simulink model "T_model_2"  (Simulink 7.2)
settings: Solver=ode23t  StartTime=0.0  StopTime=0.1  RelTol=1e-6
libraries: powerlib x19, powerlib_extras x5, srolib x3
settings Model: Creator=user  LastModifiedBy=user

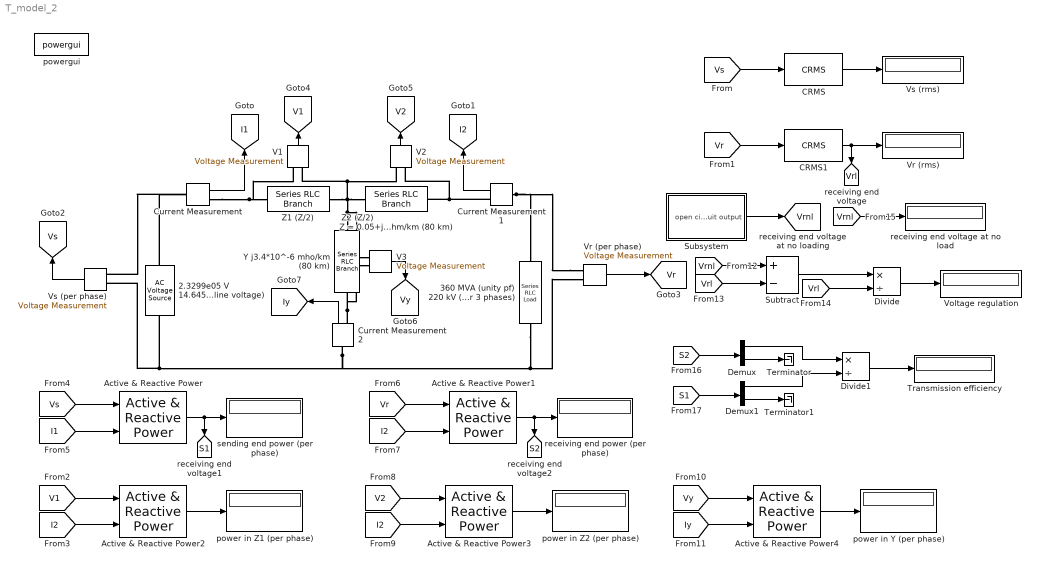
== system T_model_2 ==
  2.3299e05 V 14.64579 deg (line voltage) : powerlib/Electrical Sources/AC Voltage Source  Orientation=up  DialogController=POWERSYS.PowerSysDialog  SystemSampleTime=-1  Amplitude=(1.34526e5)*1.414  Phase=14.64579  Frequency=60  SampleTime=-1  Measurements=Voltage
  360 MVA (unity pf) 220 kV (rms) (for 3 phases) : powerlib/Elements/Series RLC Load  Orientation=down  DialogController=POWERSYS.PowerSysDialog  PhysicalDomain=powersysdomain  SubClassName=unknown  LeftPortType=p1  RightPortType=p1  LConnTagsString=a  RConnTagsString=__new0  NominalVoltage=220000/1.732  NominalFrequency=60  ActivePower=(360e6)/3  InductivePower=0  CapacitivePower=0  Setx0=off  InitialVoltage=0  SetiL0=off  InitialCurrent=0  Measurements=Branch voltage and current
  Active & Reactive Power{,1..4} (5 alike) : powerlib_extras/Measurements/Active & Reactive Power  DialogController=POWERSYS.PowerSysDialog  SystemSampleTime=-1  f1=60
  CRMS : srolib/RMS Blocks/CRMS  SystemSampleTime=-1
  CRMS1 : srolib/RMS Blocks/CRMS  SystemSampleTime=-1
  Current Measurement : powerlib/Measurements/Current Measurement  DialogController=POWERSYS.PowerSysDialog  SystemSampleTime=-1  PhasorSimulation=off  OutputType=Complex  PSBequivalent=0
  Current Measurement1 : powerlib/Measurements/Current Measurement  Orientation=left  DialogController=POWERSYS.PowerSysDialog  SystemSampleTime=-1  PhasorSimulation=off  OutputType=Complex  PSBequivalent=0
  Current Measurement2 : powerlib/Measurements/Current Measurement  Orientation=up  DialogController=POWERSYS.PowerSysDialog  SystemSampleTime=-1  PhasorSimulation=off  OutputType=Complex  PSBequivalent=0
  Demux : Demux  Outputs=2
  Demux1 : Demux  Outputs=2
  Divide : Product  Inputs=*/  OutDataType=sfix(16)  OutScaling=2^-10
  Divide1 : Product  Inputs=*/  OutDataType=sfix(16)  OutScaling=2^-10
  Subsystem : Subsystem
  Subtract : Sum  Inputs=+-  OutDataType=sfix(16)  OutScaling=2^-10
  Terminator : Terminator
  Terminator1 : Terminator
  Transmission efficiency : Display
  V1 : powerlib/Measurements/Voltage Measurement  Orientation=up  DialogController=POWERSYS.PowerSysDialog  SystemSampleTime=-1  PhasorSimulation=off  OutputType=Complex  PSBequivalent=0
  V2 : powerlib/Measurements/Voltage Measurement  Orientation=up  DialogController=POWERSYS.PowerSysDialog  SystemSampleTime=-1  PhasorSimulation=off  OutputType=Complex  PSBequivalent=0
  V3 : powerlib/Measurements/Voltage Measurement  DialogController=POWERSYS.PowerSysDialog  SystemSampleTime=-1  PhasorSimulation=off  OutputType=Complex  PSBequivalent=0
  Voltage regulation : Display
  Vr (per phase) : powerlib/Measurements/Voltage Measurement  DialogController=POWERSYS.PowerSysDialog  SystemSampleTime=-1  PhasorSimulation=off  OutputType=Complex  PSBequivalent=0
  Vr (rms) : Display
  Vs (per phase) : powerlib/Measurements/Voltage Measurement  Orientation=left  DialogController=POWERSYS.PowerSysDialog  SystemSampleTime=-1  PhasorSimulation=off  OutputType=Complex  PSBequivalent=0
  Vs (rms) : Display
  Y j3.4*10^-6 mho/km (80 km) : powerlib/Elements/Series RLC Branch  Orientation=down  DialogController=POWERSYS.PowerSysDialog  PhysicalDomain=powersysdomain  SubClassName=unknown  LeftPortType=p1  RightPortType=p1  LConnTagsString=__new0  RConnTagsString=__new0  BranchType=C  Resistance=1  Inductance=1e-3  SetiL0=off  InitialCurrent=0  Capacitance=80*(3.4e-6)/(120*3.14)  Setx0=off  InitialVoltage=0  Measurements=Branch voltage and current
  Z1 (Z/2) : powerlib/Elements/Series RLC Branch  DialogController=POWERSYS.PowerSysDialog  PhysicalDomain=powersysdomain  SubClassName=unknown  LeftPortType=p1  RightPortType=p1  LConnTagsString=__new0  RConnTagsString=__new0  BranchType=RL  Resistance=(0.05)*(80/2)  Inductance=(0.45/(120*3.14))*(80/2)  SetiL0=off  InitialCurrent=0  Capacitance=1e-6  Setx0=off  InitialVoltage=0  Measurements=Branch voltage and current
  Z2 (Z/2)                               Z = 0.05+j0.45 ohm/km (80 km) : powerlib/Elements/Series RLC Branch  DialogController=POWERSYS.PowerSysDialog  PhysicalDomain=powersysdomain  SubClassName=unknown  LeftPortType=p1  RightPortType=p1  LConnTagsString=__new0  RConnTagsString=__new0  BranchType=RL  Resistance=(0.05)*(80/2)  Inductance=(0.45/(120*3.14))*(80/2)  SetiL0=off  InitialCurrent=0  Capacitance=1e-6  Setx0=off  InitialVoltage=0  Measurements=Branch voltage and current
  power in Y (per phase) : Display
  power in Z1 (per phase) : Display
  power in Z2 (per phase) : Display
  powergui : powerlib/powergui  SystemSampleTime=-1  SimulationMode=Continuous  SampleTime=50e-6  frequency=60  SPID=off  DisableSnubberDevices=off  DisableRonSwitches=off  DisableVfSwitches=off  SwTol=0  Interpol=off  frequencyindice=60  echomessages=off  HookPort=off  FunctionMessages=off  EnableUseOfTLC=off  x0status=blocks  RestoreLinks=warning  Frange=[0:2:500]  Ylog=off  Xlog=on  ShowGrid=off  save=off  variable=ZData  ZoomFFT=on  StartTime=0.0  cycles=1  DisplayStyle=1  fundamental=60  FreqAxis=off  MaxFrequency=1000  frequencyindicesteady=1  RmsSteady=1  display=off  Ts=0  methode=off
  receiving end power (per phase) : Display
  receiving end voltage at no load : Display
  sending end power (per phase) : Display
  tag scope: I1=global, I2=global, Iy=global, S1=global, S2=global, V1=global, V2=global, Vr=global, Vrl=global, Vrnl=global, Vs=global, Vy=global
  wires:
  Vr (per phase)/1 -> [Vr]
  Current Measurement/1 -> [I1]
  Current Measurement1/1 -> [I2]
  V1/1 -> [V1]
  V2/1 -> [V2]
  V3/1 -> [Vy]
  Vs (per phase)/1 -> [Vs]
  [Vs] -> CRMS/1
  CRMS/1 -> Vs (rms)/1
  [Vr] -> CRMS1/1
  CRMS1/1 -> Vr (rms)/1, [Vrl]
  Active & Reactive Power/1 -> sending end power (per phase)/1, [S1]
  [Vs] -> Active & Reactive Power/1
  [I1] -> Active & Reactive Power/2
  Active & Reactive Power1/1 -> receiving end power (per phase)/1, [S2]
  [Vr] -> Active & Reactive Power1/1
  [I2] -> Active & Reactive Power1/2
  Active & Reactive Power2/1 -> power in Z1 (per phase)/1
  [V1] -> Active & Reactive Power2/1
  [I2] -> Active & Reactive Power2/2
  Active & Reactive Power3/1 -> power in Z2 (per phase)/1
  [V2] -> Active & Reactive Power3/1
  [I2] -> Active & Reactive Power3/2
  Active & Reactive Power4/1 -> power in Y (per phase)/1
  [Vy] -> Active & Reactive Power4/1
  [Iy] -> Active & Reactive Power4/2
  Current Measurement2/1 -> [Iy]
  Subsystem/1(open circuit output) -> [Vrnl]
  [Vrnl] -> Subtract/1
  Subtract/1 -> Divide/1
  Divide/1 -> Voltage regulation/1
  [Vrl] -> Subtract/2
  [Vrl] -> Divide/2
  [Vrnl] -> receiving end voltage at no load/1
  [S2] -> Demux/1
  Demux/2 -> Terminator/1
  [S1] -> Demux1/1
  Demux1/2 -> Terminator1/1
  Demux/1 -> Divide1/1
  Demux1/1 -> Divide1/2
  Divide1/1 -> Transmission efficiency/1
  connections:
  Vs (per phase)/LConn1 -- 2.3299e05 V 14.64579 deg (line voltage)/RConn1 -- Current Measurement/LConn1
  V1/LConn1 -- Current Measurement/RConn1 -- Z1 (Z/2)/LConn1
  Z2 (Z/2)                               Z = 0.05+j0.45 ohm/km (80 km)/LConn1 -- Y j3.4*10^-6 mho/km (80 km)/LConn1 -- V3/LConn1 -- Z1 (Z/2)/RConn1 -- V1/LConn2 -- V2/LConn1
  V2/LConn2 -- Current Measurement1/RConn1 -- Z2 (Z/2)                               Z = 0.05+j0.45 ohm/km (80 km)/RConn1
  Vr (per phase)/LConn1 -- Current Measurement1/LConn1 -- 360 MVA (unity pf) 220 kV (rms) (for 3 phases)/LConn1
  Vs (per phase)/LConn2 -- 360 MVA (unity pf) 220 kV (rms) (for 3 phases)/RConn1 -- Vr (per phase)/LConn2 -- Current Measurement2/LConn1 -- 2.3299e05 V 14.64579 deg (line voltage)/LConn1
  V3/LConn2 -- Current Measurement2/RConn1 -- Y j3.4*10^-6 mho/km (80 km)/RConn1

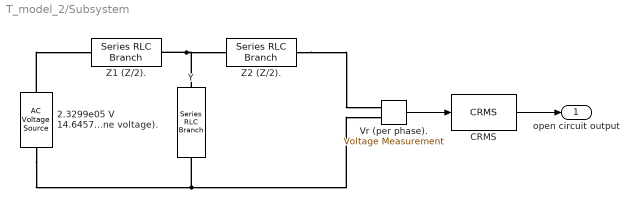
== system T_model_2/Subsystem ==
  2.3299e05 V 14.64579 deg (line voltage). : powerlib/Electrical Sources/AC Voltage Source  Orientation=up  DialogController=POWERSYS.PowerSysDialog  SystemSampleTime=-1  Amplitude=(1.34526e5)*1.414  Phase=14.64579  Frequency=60  SampleTime=-1  Measurements=Voltage
  CRMS : srolib/RMS Blocks/CRMS  SystemSampleTime=-1
  Vr (per phase). : powerlib/Measurements/Voltage Measurement  DialogController=POWERSYS.PowerSysDialog  SystemSampleTime=-1  PhasorSimulation=off  OutputType=Complex  PSBequivalent=0
  Y : powerlib/Elements/Series RLC Branch  Orientation=down  DialogController=POWERSYS.PowerSysDialog  PhysicalDomain=powersysdomain  SubClassName=unknown  LeftPortType=p1  RightPortType=p1  LConnTagsString=__new0  RConnTagsString=__new0  BranchType=C  Resistance=1  Inductance=1e-3  SetiL0=off  InitialCurrent=0  Capacitance=80*(3.4e-6)/(120*3.14)  Setx0=off  InitialVoltage=0  Measurements=Branch voltage and current
  Z1 (Z/2). : powerlib/Elements/Series RLC Branch  DialogController=POWERSYS.PowerSysDialog  PhysicalDomain=powersysdomain  SubClassName=unknown  LeftPortType=p1  RightPortType=p1  LConnTagsString=__new0  RConnTagsString=__new0  BranchType=RL  Resistance=(0.05)*(80/2)  Inductance=(0.45/(120*3.14))*(80/2)  SetiL0=off  InitialCurrent=0  Capacitance=1e-6  Setx0=off  InitialVoltage=0  Measurements=Branch voltage and current
  Z2 (Z/2). : powerlib/Elements/Series RLC Branch  DialogController=POWERSYS.PowerSysDialog  PhysicalDomain=powersysdomain  SubClassName=unknown  LeftPortType=p1  RightPortType=p1  LConnTagsString=__new0  RConnTagsString=__new0  BranchType=RL  Resistance=(0.05)*(80/2)  Inductance=(0.45/(120*3.14))*(80/2)  SetiL0=off  InitialCurrent=0  Capacitance=1e-6  Setx0=off  InitialVoltage=0  Measurements=Branch voltage and current
  open circuit output : Outport
  wires:
  Vr (per phase)./1 -> CRMS/1
  CRMS/1 -> open circuit output/1
  connections:
  2.3299e05 V 14.64579 deg (line voltage)./LConn1 -- Y/RConn1 -- Vr (per phase)./LConn2
  2.3299e05 V 14.64579 deg (line voltage)./RConn1 -- Z1 (Z/2)./LConn1
  Z2 (Z/2)./RConn1 -- Vr (per phase)./LConn1
  Y/LConn1 -- Z1 (Z/2)./RConn1 -- Z2 (Z/2)./LConn1
